simulink model "STM32_FIR_wrap"  (R2018a)
settings: Solver=FixedStepAuto  StartTime=0.0  StopTime=10.0  RelTol=1e-3  EnableMultiTasking=on
libraries: stm32f769ilib x2
settings Model: Creator=hpong  LastModifiedBy=hpong
settings OptimizationCC: EnhancedBackFolding=on  PassReuseOutputArgsAs=Individual arguments  MaxStackSize=64  OptimizeBlockOrder=speed  DifferentSizesBufferReuse=on  OptimizationCustomize=off
settings DebuggingCC: ParameterTunabilityLossMsg=error
settings HardwareCC: ProdBitPerPointer=32  ProdBitPerSizeT=32  ProdBitPerPtrDiffT=32  ProdLargestAtomicInteger=Long  ProdLargestAtomicFloat=Double  ProdWordSize=32  ProdHWDeviceType=ARM Compatible->ARM Cortex
settings SFSimCC: MATLABDynamicMemAlloc=off
settings RTWCC: SystemTargetFile=ert.tlc  HardwareBoard=STM32F769I-Discovery  TLCOptions=-aInlineSetEventsForThisBaseRateFcn=TLC_FALSE -aSuppressMultiTaskScheduler=TLC_FALSE -aRateBasedStepFcn=1  TemplateMakefile=ert_default_tmf  GenerateReport=on  Toolchain=GNU Tools for ARM Embedded Processors  IncludeHyperlinkInReport=on  LaunchReport=on  GenerateTraceInfo=on  GenerateTraceReport=on  GenerateTraceReportSl=on  GenerateTraceReportSf=on  GenerateTraceReportEml=on
settings CodeAppCC: ForceParamTrailComments=on  IgnoreCustomStorageClasses=off  OperatorAnnotations=on  SimulinkDataObjDesc=on  SFDataObjDesc=on  InsertBlockDesc=on
settings ERTTargetCC: CodeReplacementLibrary=ARM Cortex-M (CMSIS)

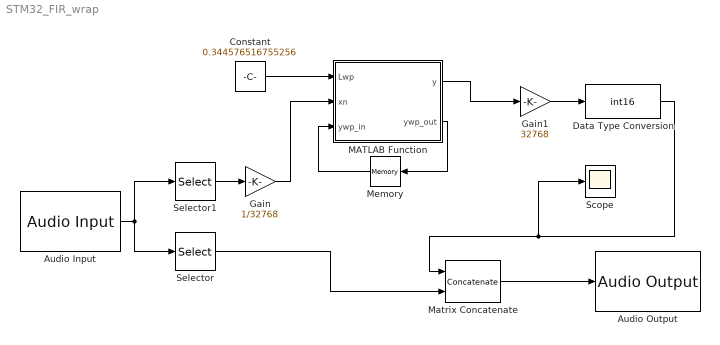
== system STM32_FIR_wrap ==
  Audio Input : stm32f769ilib/Audio Input  InputDevice=LineIn  SamplingFreq=48000  NumCh=2  FrameSize=12
      settings: SourceProductName=Embedded Coder Support Package for STMicroelectronics Discovery Boards  SourceProductBaseCode=STMICRODIS
  Audio Output : stm32f769ilib/Audio Output  OutputDevice=Headphone  SamplingFreq=48000  Volume=65
      settings: SourceProductName=Embedded Coder Support Package for STMicroelectronics Discovery Boards  SourceProductBaseCode=STMICRODIS
  Constant : Constant  Value=0.344576516755256
  Data Type Conversion : DataTypeConversion  OutDataTypeStr=int16
  Gain : Gain  Gain=1/32768  OutDataTypeStr=double
  Gain1 : Gain  Gain=32768
  MATLAB Function : MATLAB Function  TreatAsAtomicUnit=on
  Matrix Concatenate : Concatenate  Mode=Multidimensional array  ConcatenateDimension=2
  Memory : Memory  InitialCondition=[ 0 0 ; 0 0 ; 0 0 ; 0 0 ; 0 0 ; 0 0 ; 0 0 ; 0 0 ; 0 0 ; 0 0 ; 0 0 ; 0 0 ; 0 0 ; 0 0 ; 0 0 ; 0 0 ; 0 0 ; 0 0 ; 0 0 ; 0 0 ; 0 0 ; 0 0 ; 0 0 ; 0 0 ; 0 0 ; 0 0 ; 0 0 ; 0 0 ; 0 0 ; 0 0 ; 0 0 ;]  InheritSampleTime=on
  Scope : Scope
  Selector : Selector  NumberOfDimensions=2  InputPortWidth=2  IndexOptions=Select all,Index vector (dialog)  Indices=1,2  OutputSizes=1,1
  Selector1 : Selector  NumberOfDimensions=2  InputPortWidth=2  IndexOptions=Select all,Index vector (dialog)  Indices=1,1  OutputSizes=1,1
  wires:
  Matrix Concatenate/1 -> Audio Output/1
  Audio Input/1 -> Selector1/1, Selector/1
  Selector/1 -> Matrix Concatenate/2
  Selector1/1 -> Gain/1
  Gain1/1 -> Data Type Conversion/1
  MATLAB Function/1(y) -> Gain1/1
  Data Type Conversion/1 -> Scope/1, Matrix Concatenate/1
  Constant/1 -> MATLAB Function/1(Lwp)
  MATLAB Function/2(ywp_out) -> Memory/1
  Memory/1 -> MATLAB Function/3(ywp_in)
  Gain/1 -> MATLAB Function/2(xn)

== matlab function STM32_FIR_wrap/MATLAB Function ==
  data: Lwp input; xn input; y output; ywp_in input; ywp_out output
function [y, ywp_out] = fir_wrap(Lwp,xn, ywp_in)
b = [0.00000000  0.00120143  0.00278433  0.00422732  0.00394276  -0.00000000  -0.00825678  -0.01858321  -0.02538982  -0.02123531  0.00000000  0.03958811  0.09188888  0.14509908  0.18490288  0.19966067  0.18490288  0.14509908  0.09188888  0.03958811  0.00000000  -0.02123531  -0.02538982  -0.01858321  -0.00825678  -0.00000000  0.00394276  0.00422732  0.00278433  0.00120143  0.00000000  ];
nb = length(b);
y=ones(12,1,'double');
ywp = ywp_in;
xm = [ywp_in(nb,1) ;xn]; %4*1
for n=2:13
    ywp(1,2) = ywp(1,1);
    ywp(1,1) = (ywp(1,2)-xm(n))*Lwp + xm(n-1);
    y(n-1)=b(1)*xm(n) + b(2)*ywp(1,1); 
    for nn=2:nb-1
        ywp(nn,2) = ywp(nn,1);
        ywp(nn,1) = (ywp(nn,2)-ywp(nn-1,1))*Lwp + ywp(nn-1,2);
        y(n-1) = y(n-1) + b(nn+1)*ywp(nn,1);
    end
end
ywp_out = ywp;
ywp_out(nb,1) = xm(13);
end
